simulink model "simulink_A2_Final"  (R2023a)
settings: Solver=FixedStepAuto  StartTime=0.0  StopTime=30  FixedStep=1e-3  RelTol=1e-3  EnableMultiTasking=on
undefined symbols (not defined in the file): A0, A1, D0, D1, D10, D11, D12, D13, D2, D3, D4, D5, D6, D7, D8, D9, PTA0, PTA1, PTA2, PTB2, PTB23, PTB3, PTB9, PTC16, PTC17, PTC2, PTC3, PTC4, PTD0, PTD1, PTD2, PTD3
libraries: etargetslib x24, frdmk64flib x20, dspstat3 x1
settings Model: ExtModeTrigDuration=5  Creator=Karm  LastModifiedBy=lison
settings OptimizationCC: EnhancedBackFolding=on  PassReuseOutputArgsAs=Individual arguments  ZeroExternalMemoryAtStartup=off  ZeroInternalMemoryAtStartup=off  MaxStackSize=64  OptimizeBlockOrder=speed  DifferentSizesBufferReuse=on  OptimizationCustomize=off  EfficientTunableParamExpr=on
settings DebuggingCC: ParameterPrecisionLossMsg=none  ParameterTunabilityLossMsg=error
settings HardwareCC: ProdBitPerPointer=32  ProdBitPerSizeT=32  ProdBitPerPtrDiffT=32  ProdLargestAtomicInteger=Long  ProdLargestAtomicFloat=Double  ProdWordSize=32  ProdHWDeviceType=ARM Compatible->ARM Cortex
settings SFSimCC: MATLABDynamicMemAlloc=off
settings RTWCC: Description=Embedded Coder  SystemTargetFile=ert.tlc  HardwareBoard=NXP FRDM-K64F  TLCOptions="-aInlineSetEventsForThisBaseRateFcn=TLC_FALSE -aSuppressMultiTaskScheduler=TLC_FALSE  -aRateBasedStepFcn=0"  TemplateMakefile=ert_default_tmf  Toolchain=GNU Tools for ARM Embedded Processors
settings CodeAppCC: ForceParamTrailComments=on  IgnoreCustomStorageClasses=off  OperatorAnnotations=on  SimulinkDataObjDesc=on  SFDataObjDesc=on  InsertBlockDesc=on
settings ERTTargetCC: ExtModeTransport=4  ExtModeMexFile=sendToCommService

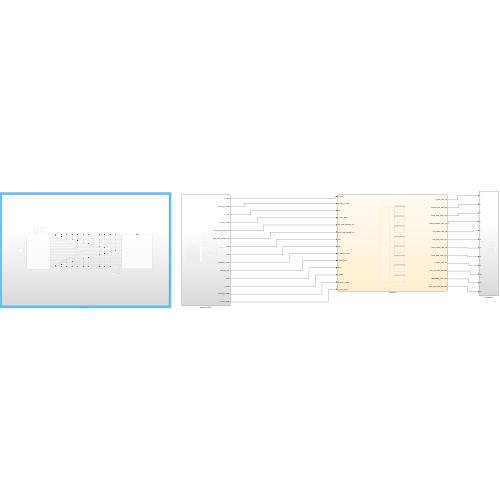
[thumbnail: Simulink's stored preview of the top-level diagram]
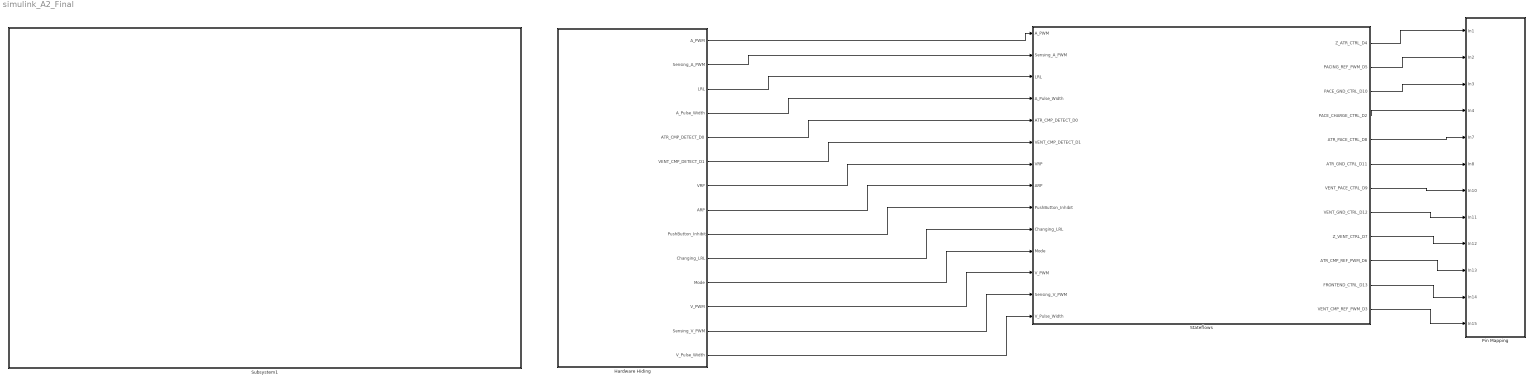
== system simulink_A2_Final ==
  Hardware Hiding : Subsystem
  Pin Mapping : Subsystem
  Stateflows : Stateflow chart  TreatAsAtomicUnit=on
      settings: PortSchema="{\"entries\":[{\"content\":{\"sides\":[{\"content\":{\"connectorIds\":[\"In1\",\"In9\",\"In2\",\"In8\",\"In3\",\"In4\",\"In5\",\"In6\",\"In7\",\"In10\",\"In11\",\"In12\",\"In13\",\"In14\"]},\"type\":\"ConnectorPlacement.EquallySpacedRectSide\",\"uuid\":\"fd7a65b5-6a9e-486c-b395-8752d247d110\"},{\"content\":{\"connectorIds\":[\"Out1\",\"Out2\",\"Out3\",\"Out4\",\"Out5\",\"Out6\",\"Out7\",\"Out8\",\"Out9\",\"Out10\",\"Out11\",\"Out12\"],\"side\":\"RIGHT\"},\"type\":\"ConnectorPlacement.EquallySpacedRectSide\",\"uuid\":\"2771a934-b7e6-4717-9d0f-b17bdbdca872\"},{\"content\":{\"side\":\"TOP\"},\"type\":\"ConnectorPlacement.EquallySpacedRectSide\",\"uuid\":\"3a68066b-1574-4876-94b5-372b67bc25b8\"}]},\"type\":\"ConnectorPlacement.EquallySpacedConnector\",\"uuid\":\"cd95133d-7553-4814-ba78-1fbdc0c00507\"}],\"packageUris\":[\"http://schema.mathworks.com/mf0/Connector/R2020b\"],\"version\":\"1.0\"}"
  Subsystem1 : Subsystem
  wires:
  Hardware Hiding/1(A_PWM) -> Stateflows/1(A_PWM)
  Hardware Hiding/2(Sensing_A_PWM) -> Stateflows/9(Sensing_A_PWM)
  Hardware Hiding/3(LRL) -> Stateflows/2(LRL)
  Hardware Hiding/4(A_Pulse_Width) -> Stateflows/8(A_Pulse_Width)
  Hardware Hiding/5(ATR_CMP_DETECT_D0) -> Stateflows/3(ATR_CMP_DETECT_D0)
  Hardware Hiding/6(VENT_CMP_DETECT_D1) -> Stateflows/4(VENT_CMP_DETECT_D1)
  Hardware Hiding/7(VRP) -> Stateflows/5(VRP)
  Hardware Hiding/8(ARP) -> Stateflows/6(ARP)
  Hardware Hiding/9(PushButton_Inhibit) -> Stateflows/7(PushButton_Inhibit)
  Stateflows/1(Z_ATR_CTRL_D4) -> Pin Mapping/1(In1)
  Stateflows/2(PACING_REF_PWM_D5) -> Pin Mapping/2(In2)
  Stateflows/3(PACE_GND_CTRL_D10) -> Pin Mapping/3(In3)
  Stateflows/4(PACE_CHARGE_CTRL_D2) -> Pin Mapping/4(In4)
  Stateflows/5(ATR_PACE_CTRL_D8) -> Pin Mapping/5(In7)
  Stateflows/6(ATR_GND_CTRL_D11) -> Pin Mapping/6(In8)
  Stateflows/7(VENT_PACE_CTRL_D9) -> Pin Mapping/7(In10)
  Stateflows/8(VENT_GND_CTRL_D12) -> Pin Mapping/8(In11)
  Stateflows/9(Z_VENT_CTRL_D7) -> Pin Mapping/9(In12)
  Stateflows/10(ATR_CMP_REF_PWM_D6) -> Pin Mapping/10(In13)
  Stateflows/11(FRONTEND_CTRL_D13) -> Pin Mapping/11(In14)
  Stateflows/12(VENT_CMP_REF_PWM_D3) -> Pin Mapping/12(In15)
  Hardware Hiding/10(Changing_LRL) -> Stateflows/10(Changing_LRL)
  Hardware Hiding/11(Mode) -> Stateflows/11(Mode)
  Hardware Hiding/12(V_PWM) -> Stateflows/12(V_PWM)
  Hardware Hiding/13(Sensing_V_PWM) -> Stateflows/13(Sensing_V_PWM)
  Hardware Hiding/14(V_Pulse_Width) -> Stateflows/14(V_Pulse_Width)

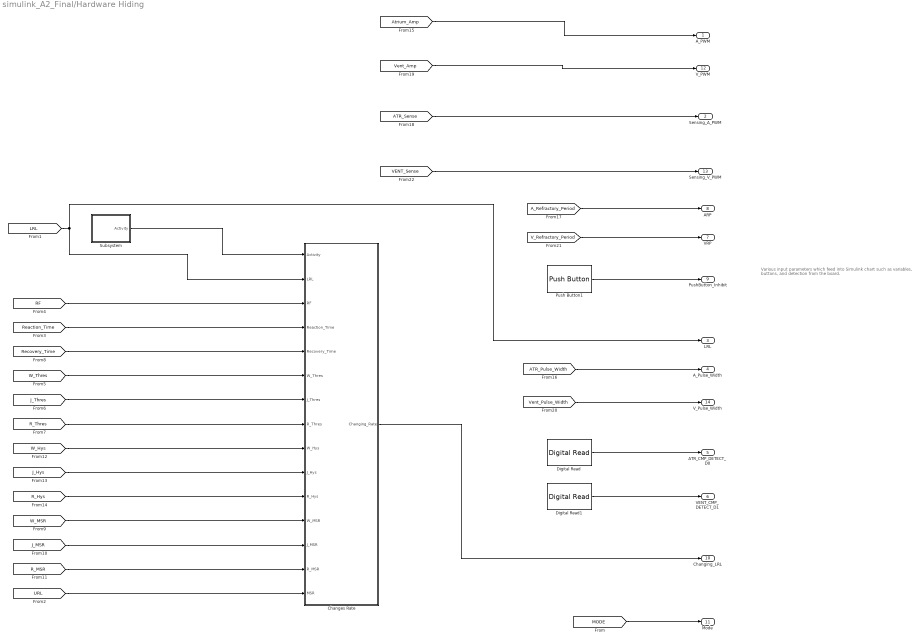
== system simulink_A2_Final/Hardware Hiding ==
  note: Various input parameters which feed into
      | Simulink chart such as variables, buttons, and
      | detection from the board.
  Changes Rate : Stateflow chart  TreatAsAtomicUnit=on
  Digital Read : frdmk64flib/Digital Read  Whichpin=PTC16 (D0)  SampleTime=-1
  Digital Read1 : frdmk64flib/Digital Read  Whichpin=PTC17 (D1)  SampleTime=-1
  Push Button1 : frdmk64flib/Push Button  Whichswitch=SW3  SampleTime1=-1
  Subsystem : Subsystem
  A_PWM : Outport  OutDataTypeStr=single
  Sensing_A_PWM : Outport  Port=2  OutDataTypeStr=single
  LRL : Outport  Port=3  OutDataTypeStr=uint16
  A_Pulse_Width : Outport  Port=4  OutDataTypeStr=uint16
  ATR_CMP_DETECT_D0 : Outport  Port=5
  VENT_CMP_DETECT_D1 : Outport  Port=6
  VRP : Outport  Port=7  OutDataTypeStr=uint16
  ARP : Outport  Port=8  OutDataTypeStr=uint16
  PushButton_Inhibit : Outport  Port=9
  Changing_LRL : Outport  Port=10  OutDataTypeStr=uint16
  Mode : Outport  Port=11  OutDataTypeStr=uint8
  V_PWM : Outport  Port=12  OutDataTypeStr=single
  Sensing_V_PWM : Outport  Port=13
  V_Pulse_Width : Outport  Port=14  OutDataTypeStr=uint16
  wires:
  Push Button1/1 -> PushButton_Inhibit/1
  [V_Refractory_Period] -> VRP/1
  [A_Refractory_Period] -> ARP/1
  [LRL] -> LRL/1, Changes Rate/2(LRL)
  [ATR_Pulse_Width] -> A_Pulse_Width/1
  Digital Read/1 -> ATR_CMP_DETECT_D0/1
  Digital Read1/1 -> VENT_CMP_DETECT_D1/1
  [W_Thres] -> Changes Rate/6(W_Thres)
  [RF] -> Changes Rate/3(RF)
  [Recovery_Time] -> Changes Rate/5(Recovery_Time)
  [J_Thres] -> Changes Rate/7(J_Thres)
  [R_Thres] -> Changes Rate/8(R_Thres)
  [W_Hys] -> Changes Rate/9(W_Hys)
  [J_Hys] -> Changes Rate/10(J_Hys)
  [R_Hys] -> Changes Rate/11(R_Hys)
  [W_MSR] -> Changes Rate/12(W_MSR)
  [J_MSR] -> Changes Rate/13(J_MSR)
  [R_MSR] -> Changes Rate/14(R_MSR)
  Subsystem/1(Activity) -> Changes Rate/1(Activity)
  [Reaction_Time] -> Changes Rate/4(Reaction_Time)
  Changes Rate/1(Changing_Rate) -> Changing_LRL/1
  [URL] -> Changes Rate/15(MSR)
  [MODE] -> Mode/1
  [Vent_Pulse_Width] -> V_Pulse_Width/1
  [VENT_Sense] -> Sensing_V_PWM/1
  [ATR_Sense] -> Sensing_A_PWM/1
  [Vent_Amp] -> V_PWM/1
  [Atrium_Amp] -> A_PWM/1

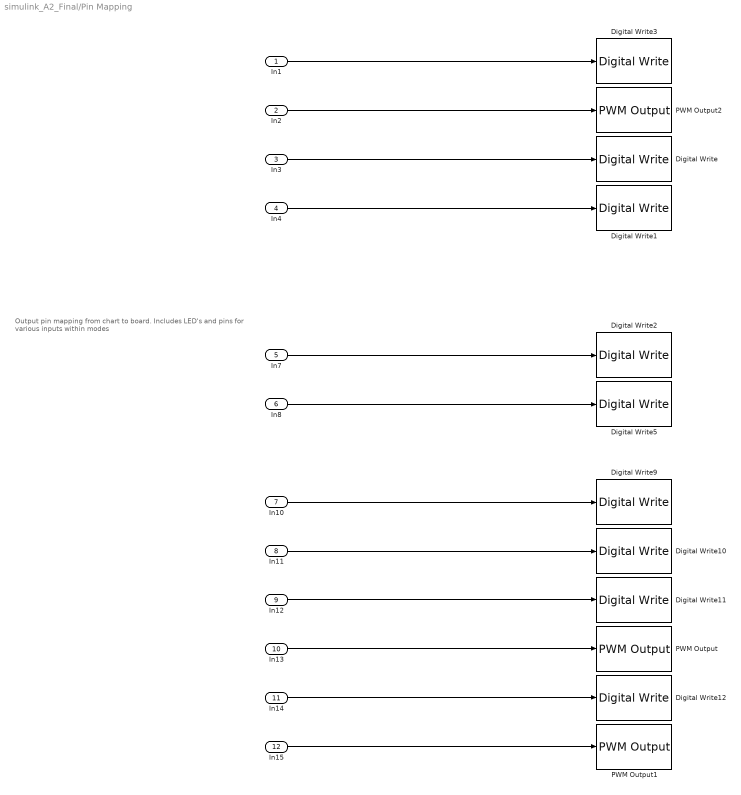
== system simulink_A2_Final/Pin Mapping ==
  note: Output pin mapping from chart to board.
      | Includes LED's and pins for various
      | inputs within modes
  In1 : Inport
  In2 : Inport  Port=2
  In3 : Inport  Port=3
  In4 : Inport  Port=4
  In7 : Inport  Port=5
  In8 : Inport  Port=6
  In10 : Inport  Port=7
  In11 : Inport  Port=8
  In12 : Inport  Port=9
  In13 : Inport  Port=10
  In14 : Inport  Port=11
  In15 : Inport  Port=12
  Digital Write : frdmk64flib/Digital Write  Whichpin=PTD0 (D10)
  Digital Write1 : frdmk64flib/Digital Write  Whichpin=PTB9 (D2)
  Digital Write10 : frdmk64flib/Digital Write  Whichpin=PTD3 (D12)
  Digital Write11 : frdmk64flib/Digital Write  Whichpin=PTC3 (D7)
  Digital Write12 : frdmk64flib/Digital Write  Whichpin=PTD1 (D13)
  Digital Write2 : frdmk64flib/Digital Write  Whichpin=PTA0 (D8)
  Digital Write3 : frdmk64flib/Digital Write  Whichpin=PTB23 (D4)
  Digital Write5 : frdmk64flib/Digital Write  Whichpin=PTD2 (D11)
  Digital Write9 : frdmk64flib/Digital Write  Whichpin=PTC4 (D9)
  PWM Output : frdmk64flib/PWM Output  Whichpin=PTC2 (D6)  InitialFrequency=2000  InitialDutyCycle=0
  PWM Output1 : frdmk64flib/PWM Output  Whichpin=PTA1 (D3)  InitialFrequency=2000  InitialDutyCycle=0
  PWM Output2 : frdmk64flib/PWM Output  Whichpin=PTA2 (D5)  InitialFrequency=2000  InitialDutyCycle=0
  wires:
  In1/1 -> Digital Write3/1
  In2/1 -> PWM Output2/1
  In4/1 -> Digital Write1/1
  In8/1 -> Digital Write5/1
  In7/1 -> Digital Write2/1
  In3/1 -> Digital Write/1
  In12/1 -> Digital Write11/1
  In10/1 -> Digital Write9/1
  In11/1 -> Digital Write10/1
  In13/1 -> PWM Output/1
  In15/1 -> PWM Output1/1
  In14/1 -> Digital Write12/1

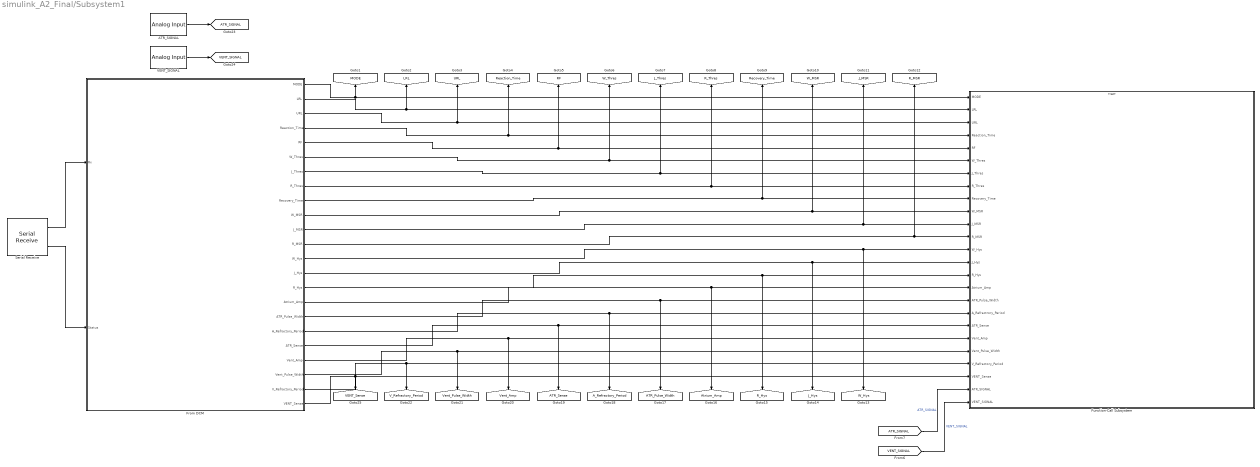
== system simulink_A2_Final/Subsystem1 ==
  ATR_SIGNAL : frdmk64flib/Analog Input  Whichpin=PTB2 (A0)  SampleTime=-1
  From DCM : Stateflow chart  TreatAsAtomicUnit=on
      settings: PortSchema="{\"entries\":[{\"content\":{\"sides\":[{\"content\":{\"connectorIds\":[\"In1\",\"In2\"]},\"type\":\"ConnectorPlacement.EquallySpacedRectSide\",\"uuid\":\"cf186c72-5509-48fa-91bf-627d929b9ac9\"},{\"content\":{\"connectorIds\":[\"Out3\",\"Out1\",\"Out2\",\"Out4\",\"Out5\",\"Out6\",\"Out7\",\"Out8\",\"Out9\",\"Out10\",\"Out11\",\"Out12\",\"Out13\",\"Out14\",\"Out15\",\"Out16\",\"Out17\",\"Out18\",\"Out19\",\"Out20\",\"Out21\",\"Out22\",\"Out23\"],\"side\":\"RIGHT\"},\"type\":\"ConnectorPlacement.EquallySpacedRectSide\",\"uuid\":\"f11b7b65-e2af-422d-8d59-d5e19782ba77\"},{\"content\":{\"side\":\"TOP\"},\"type\":\"ConnectorPlacement.EquallySpacedRectSide\",\"uuid\":\"83f5ca47-954b-473f-a694-ccb4a0a9db86\"},{\"content\":{\"side\":\"BOTTOM\"},\"type\":\"ConnectorPlacement.EquallySpacedRectSide\",\"uuid\":\"1b259bf9-85ed-487d-ae78-9bbf0cb8bebe\"}]},\"type\":\"ConnectorPlacement.EquallySpacedConnector\",\"uuid\":\"33095ea8-75ce-40a2-933c-32919530d49f\"}],\"packageUris\":[\"http://schema.mathworks.com/mf0/Connector/R2020b\"],\"version\":\"1.0\"}"
  Function-Call Subsystem : Subsystem  TreatAsAtomicUnit=on
  Serial Receive : frdmk64flib/Serial Receive  SCIModule=0  Baudrate=uint32(9600)  Parity=None  StopBits=1  HardwareFlowControl=None  ByteOrder=LittleEndian  DataType=uint8  DataLength=91  BlockingMode=off  OutputStatus=on  SampleTime=-1
  VENT_SIGNAL : frdmk64flib/Analog Input  Whichpin=PTB3 (A1)  SampleTime=-1
  tag scope: ATR_Pulse_Width=global, ATR_SIGNAL=global, ATR_Sense=global, A_Refractory_Period=global, Atrium_Amp=global, J_Hys=global, J_MSR=global, J_Thres=global, LRL=global, MODE=global, RF=global, R_Hys=global, R_MSR=global, R_Thres=global, Reaction_Time=global, Recovery_Time=global, URL=global, VENT_SIGNAL=global, VENT_Sense=global, V_Refractory_Period=global, Vent_Amp=global, Vent_Pulse_Width=global, W_Hys=global, W_MSR=global, W_Thres=global
  wires:
  Serial Receive/2 -> From DCM/2(Status)
  Serial Receive/1 -> From DCM/1(Rx)
  From DCM/3(MODE) -> Function-Call Subsystem/1(MODE), [MODE]
  From DCM/1(LRL) -> Function-Call Subsystem/2(LRL), [LRL]
  From DCM/2(URL) -> Function-Call Subsystem/3(URL), [URL]
  From DCM/4(Reaction_Time) -> Function-Call Subsystem/4(Reaction_Time), [Reaction_Time]
  From DCM/5(RF) -> Function-Call Subsystem/5(RF), [RF]
  From DCM/6(W_Thres) -> Function-Call Subsystem/6(W_Thres), [W_Thres]
  From DCM/7(J_Thres) -> Function-Call Subsystem/7(J_Thres), [J_Thres]
  From DCM/8(R_Thres) -> Function-Call Subsystem/8(R_Thres), [R_Thres]
  From DCM/9(Recovery_Time) -> Function-Call Subsystem/9(Recovery_Time), [Recovery_Time]
  From DCM/10(W_MSR) -> Function-Call Subsystem/10(W_MSR), [W_MSR]
  From DCM/11(J_MSR) -> Function-Call Subsystem/11(J_MSR), [J_MSR]
  From DCM/12(R_MSR) -> Function-Call Subsystem/12(R_MSR), [R_MSR]
  From DCM/13(W_Hys) -> Function-Call Subsystem/13(W_Hys), [W_Hys]
  From DCM/14(J_Hys) -> Function-Call Subsystem/14(J_Hys), [J_Hys]
  From DCM/15(R_Hys) -> Function-Call Subsystem/15(R_Hys), [R_Hys]
  From DCM/16(Atrium_Amp) -> Function-Call Subsystem/16(Atrium_Amp), [Atrium_Amp]
  From DCM/17(ATR_Pulse_Width) -> Function-Call Subsystem/17(ATR_Pulse_Width), [ATR_Pulse_Width]
  From DCM/18(A_Refractory_Period) -> Function-Call Subsystem/18(A_Refractrory_Period), [A_Refractory_Period]
  From DCM/19(ATR_Sense) -> Function-Call Subsystem/19(ATR_Sense), [ATR_Sense]
  From DCM/21(Vent_Pulse_Width) -> Function-Call Subsystem/21(Vent_Pulse_Width), [Vent_Pulse_Width]
  From DCM/22(V_Refractory_Period) -> Function-Call Subsystem/22(V_Refractory_Period), [V_Refractory_Period]
  From DCM/23(VENT_Sense) -> Function-Call Subsystem/23(VENT_Sense), [VENT_Sense]
  ATR_SIGNAL/1 -> [ATR_SIGNAL]
  VENT_SIGNAL/1 -> [VENT_SIGNAL]
  From DCM/20(Vent_Amp) -> Function-Call Subsystem/20(Vent_Amp), [Vent_Amp]
  [ATR_SIGNAL] -> Function-Call Subsystem/24(ATR_SIGNAL)  "ATR_SIGNAL"
  [VENT_SIGNAL] -> Function-Call Subsystem/25(VENT_SIGNAL)  "VENT_SIGNAL"

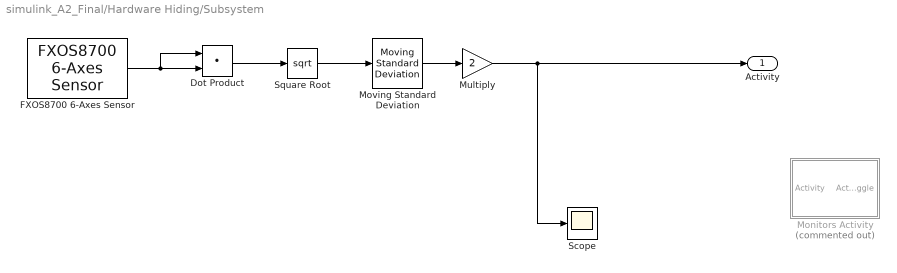
== system simulink_A2_Final/Hardware Hiding/Subsystem ==
  Dot Product : DotProduct  OutDataTypeStr=Inherit: Inherit via internal rule
  FXOS8700 6-Axes Sensor : frdmk64flib/FXOS8700 6-Axes Sensor  Activesensor=Accelerometer only  ODR=800Hz  HybridODR=400Hz  Accelfullrange=-4g to +4g  SampleTime=-1
  Monitors Activity : Stateflow chart  Commented=on  TreatAsAtomicUnit=on
  Moving Standard Deviation : dspstat3/Moving Standard Deviation  Method=Sliding window  ForgettingFactorPort=off  SpecifyWindowLength=on  WindowLength=4  OverlapLength=3  AllowArbitraryInputLength=off  ForgettingFactor=0.9  SimulateUsing=Code generation
  Multiply : Gain  Gain=2
  Scope : Scope
  Square Root : Sqrt
  Activity : Outport
  wires:
  Square Root/1 -> Moving Standard Deviation/1
  Moving Standard Deviation/1 -> Multiply/1
  Dot Product/1 -> Square Root/1
  FXOS8700 6-Axes Sensor/1 -> Dot Product/2, Dot Product/1
  Multiply/1 -> Scope/1, Activity/1

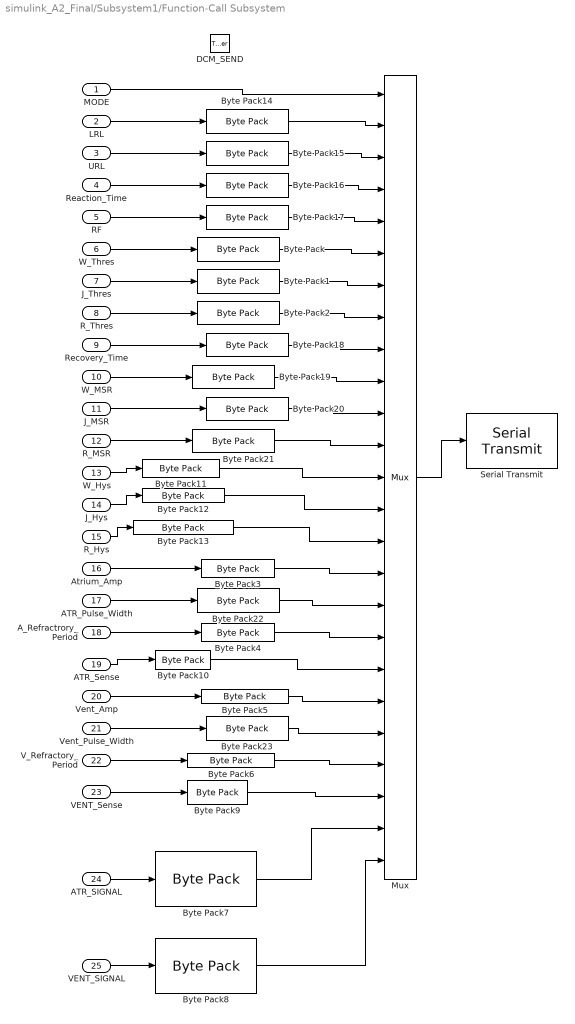
== system simulink_A2_Final/Subsystem1/Function-Call Subsystem ==
  MODE : Inport  OutDataTypeStr=uint8
  LRL : Inport  Port=2  OutDataTypeStr=uint16
  URL : Inport  Port=3  OutDataTypeStr=uint16
  Reaction_Time : Inport  Port=4  OutDataTypeStr=uint16
  RF : Inport  Port=5  OutDataTypeStr=uint16
  W_Thres : Inport  Port=6  OutDataTypeStr=double
  J_Thres : Inport  Port=7  OutDataTypeStr=double
  R_Thres : Inport  Port=8  OutDataTypeStr=double
  Recovery_Time : Inport  Port=9  OutDataTypeStr=uint16
  W_MSR : Inport  Port=10  OutDataTypeStr=uint16
  J_MSR : Inport  Port=11  OutDataTypeStr=uint16
  R_MSR : Inport  Port=12  OutDataTypeStr=uint16
  W_Hys : Inport  Port=13  OutDataTypeStr=double
  J_Hys : Inport  Port=14  OutDataTypeStr=double
  R_Hys : Inport  Port=15  OutDataTypeStr=double
  Atrium_Amp : Inport  Port=16  OutDataTypeStr=single
  ATR_Pulse_Width : Inport  Port=17  OutDataTypeStr=uint16
  A_Refractrory_Period : Inport  Port=18  OutDataTypeStr=uint16
  ATR_Sense : Inport  Port=19  OutDataTypeStr=single
  Vent_Amp : Inport  Port=20  OutDataTypeStr=single
  Vent_Pulse_Width : Inport  Port=21  OutDataTypeStr=uint16
  V_Refractory_Period : Inport  Port=22  OutDataTypeStr=uint16
  VENT_Sense : Inport  Port=23  OutDataTypeStr=single
  ATR_SIGNAL : Inport  Port=24  OutDataTypeStr=double
  VENT_SIGNAL : Inport  Port=25  OutDataTypeStr=double
  DCM_SEND : TriggerPort  TriggerType=function-call  IsSimulinkFunction=on  FunctionName=DCM_SEND  VariantControl=(inherit)
  Byte Pack{,1..2,7..8,11..13} (8 alike) : etargetslib/Byte Pack  datatypes={'double'}  byteAlign=1
  Byte Pack{3,5,9..10} (4 alike) : etargetslib/Byte Pack  datatypes={'single'}  byteAlign=1
  Byte Pack{4,6,14..23} (12 alike) : etargetslib/Byte Pack  datatypes={'uint16'}  byteAlign=1
  Mux : Mux  Inputs=25
  Serial Transmit : frdmk64flib/Serial Transmit  SCIModule=0  Baudrate=uint32(9600)  Parity=None  StopBits=1  HardwareFlowControl=None  ByteOrder=LittleEndian  BlockingMode=on  OutputStatus=off
  wires:
  MODE/1 -> Mux/1
  Reaction_Time/1 -> Byte Pack16/1
  RF/1 -> Byte Pack17/1
  W_Thres/1 -> Byte Pack/1
  Byte Pack/1 -> Mux/6
  J_Thres/1 -> Byte Pack1/1
  Byte Pack1/1 -> Mux/7
  Recovery_Time/1 -> Byte Pack18/1
  R_Thres/1 -> Byte Pack2/1
  Byte Pack2/1 -> Mux/8
  W_MSR/1 -> Byte Pack19/1
  J_MSR/1 -> Byte Pack20/1
  R_MSR/1 -> Byte Pack21/1
  Atrium_Amp/1 -> Byte Pack3/1
  ATR_Pulse_Width/1 -> Byte Pack22/1
  Byte Pack3/1 -> Mux/16
  A_Refractrory_Period/1 -> Byte Pack4/1
  Byte Pack4/1 -> Mux/18
  Vent_Amp/1 -> Byte Pack5/1
  Byte Pack5/1 -> Mux/20
  Vent_Pulse_Width/1 -> Byte Pack23/1
  V_Refractory_Period/1 -> Byte Pack6/1
  Byte Pack6/1 -> Mux/22
  Mux/1 -> Serial Transmit/1
  ATR_SIGNAL/1 -> Byte Pack7/1
  Byte Pack7/1 -> Mux/24
  VENT_SIGNAL/1 -> Byte Pack8/1
  Byte Pack8/1 -> Mux/25
  VENT_Sense/1 -> Byte Pack9/1
  Byte Pack9/1 -> Mux/23
  ATR_Sense/1 -> Byte Pack10/1
  Byte Pack10/1 -> Mux/19
  W_Hys/1 -> Byte Pack11/1
  Byte Pack11/1 -> Mux/13
  J_Hys/1 -> Byte Pack12/1
  Byte Pack12/1 -> Mux/14
  R_Hys/1 -> Byte Pack13/1
  Byte Pack13/1 -> Mux/15
  LRL/1 -> Byte Pack14/1
  Byte Pack14/1 -> Mux/2
  URL/1 -> Byte Pack15/1
  Byte Pack15/1 -> Mux/3
  Byte Pack16/1 -> Mux/4
  Byte Pack17/1 -> Mux/5
  Byte Pack18/1 -> Mux/9
  Byte Pack19/1 -> Mux/10
  Byte Pack20/1 -> Mux/11
  Byte Pack21/1 -> Mux/12
  Byte Pack22/1 -> Mux/17
  Byte Pack23/1 -> Mux/21

== stateflow chart simulink_A2_Final/Hardware Hiding/Subsystem/Monitors Activity ==
  state entry
    if Activity > 1.0
    Act_Toggle = true;
    else
    Act_Toggle = false;
    end
  (default) -> entry
  data: Activity input; Act_Toggle output

== stateflow chart simulink_A2_Final/Stateflows ==
  state Start
  state VOO
    state Charging
      % parameters laid out by documentation for Charging
      entry:
      PACING_REF_PWM_D5 = (V_PWM/5)*100;
      PACE_GND_CTRL_D10 = 1;
      VENT_GND_CTRL_D12 = 1;
      PACE_CHARGE_CTRL_D2 = 1;
      Z_VENT_CTRL_D7 = 0;
      VENT_PACE_CTRL_D9 = 0;
      Pulse_Period = (60000/LRL);
    state Pacing
      % parameters laid out by documentation for Pacing
      entry:
      PACING_REF_PWM_D5 = (V_PWM/5)*100;
      VENT_PACE_CTRL_D9 = 1;
      VENT_GND_CTRL_D12 = 0;
      PACE_CHARGE_CTRL_D2 = 0;
      PACE_GND_CTRL_D10 = 1;
      Z_VENT_CTRL_D7 = 0;
    note: Ventricular pacing, no sensing
    (default) -> VOO.Charging
    VOO.Charging -> VOO.Pacing : [after(Pulse_Period-V_Pulse_Width,msec)]
    VOO.Pacing -> VOO.Charging : [after(V_Pulse_Width,msec)]
  state VVI
    note: Ventricular pacing, ventricular sensing, sensed intrinsic signal inhibits ventricular pacing
    state Pacing2
      % parameters laid out by documentation for Pacing
      entry:
      PACE_CHARGE_CTRL_D2 = 0;
      PACE_GND_CTRL_D10 = 1;
      Z_VENT_CTRL_D7 = 0;
      VENT_GND_CTRL_D12 = 0;
      VENT_PACE_CTRL_D9 = 1;
    state Charging2
      % parameters laid out by documentation for Charging
      entry:
      FRONTEND_CTRL_D13 = 1;
      VENT_CMP_REF_PWM_D3 = (Sensing_V_PWM/5)*100;
      PACING_REF_PWM_D5 = (V_PWM/5)*100;
      VENT_PACE_CTRL_D9 = 0;
      PACE_CHARGE_CTRL_D2 = 1;
      PACE_GND_CTRL_D10 = 1;
      Z_VENT_CTRL_D7 = 0;
      VENT_GND_CTRL_D12 = 1;
      Pulse_Period = (60000/LRL);
    state Refractor_and_Sensing
    (default) -> VVI.Charging2
    VVI.Pacing2 -> VVI.Charging2 : [after(V_Pulse_Width,msec)]
    VVI.Refractor_and_Sensing -> VVI.Pacing2 [order 2] : after(Pulse_Period-VRP-V_Pulse_Width,msec)[VENT_CMP_DETECT_D1 == 0 & PushButton_Inhibit == false]
    VVI.Charging2 -> VVI.Refractor_and_Sensing : after(VRP,msec)
    VVI.Refractor_and_Sensing -> VVI.Charging2 [order 1] : [VENT_CMP_DETECT_D1 == 1 | PushButton_Inhibit == true]
  state AOO
    note: Atrial pacing, no sensing
    state Charging1
      % parameters laid out by documentation for Charging
      entry:
      PACING_REF_PWM_D5 = (A_PWM/5)*100;
      PACE_CHARGE_CTRL_D2 = 1;
      ATR_PACE_CTRL_D8 = 0;
      PACE_GND_CTRL_D10 = 1;
      ATR_GND_CTRL_D11 = 1;
      Z_ATR_CTRL_D4 = 0;
      Pulse_Period = (60000/LRL);
    state Pacing1
      % parameters laid out by documentation for Pacing
      entry:
      PACING_REF_PWM_D5 = (A_PWM/5)*100;
      PACE_CHARGE_CTRL_D2 = 0;
      PACE_GND_CTRL_D10 = 1;
      ATR_PACE_CTRL_D8 = 1;
      ATR_GND_CTRL_D11 = 0;
      Z_ATR_CTRL_D4 = 0;
    (default) -> AOO.Charging1
    AOO.Charging1 -> AOO.Pacing1 : [after(Pulse_Period-A_Pulse_Width,msec)]
    AOO.Pacing1 -> AOO.Charging1 : [after(A_Pulse_Width,msec)]
  state AAI
    state Pacing3
      % parameters laid out by documentation for Pacing
      entry:
      PACING_REF_PWM_D5 = (A_PWM/5)*100;
      PACE_CHARGE_CTRL_D2=0;
      ATR_PACE_CTRL_D8= 1;
      ATR_GND_CTRL_D11= 0;
      PACE_GND_CTRL_D10=1;
      Z_ATR_CTRL_D4=0;
    state Charging3
      % parameters laid out by documentation for Charging
      entry:
      PACING_REF_PWM_D5 = (A_PWM/5)*100;
      PACE_CHARGE_CTRL_D2=1;
      ATR_PACE_CTRL_D8= 0;
      ATR_GND_CTRL_D11= 1;
      PACE_GND_CTRL_D10=1;
      Z_ATR_CTRL_D4=0;
      FRONTEND_CTRL_D13 = 1;
      ATR_CMP_REF_PWM_D6 = (Sensing_A_PWM/5)*100;
      Pulse_Period = (60000/LRL);
    state Refractor_and_Sensing
    note: Atrial pacing, atrial sensing, sensed intrinsic signal inhibits atrial pacing
    (default) -> AAI.Charging3
    AAI.Refractor_and_Sensing -> AAI.Charging3 [order 1] : [ATR_CMP_DETECT_D0 == 1 | PushButton_Inhibit == true]
    AAI.Refractor_and_Sensing -> AAI.Pacing3 [order 2] : after(Pulse_Period-ARP-A_Pulse_Width,msec)[ATR_CMP_DETECT_D0 == 0 & PushButton_Inhibit == false]
    AAI.Charging3 -> AAI.Refractor_and_Sensing : after(ARP, msec)
    AAI.Pacing3 -> AAI.Charging3 : after(A_Pulse_Width,msec)
  state VOOR
    state Charging
      % parameters laid out by documentation for Charging
      entry:
      PACING_REF_PWM_D5 = (V_PWM/5)*100;
      PACE_CHARGE_CTRL_D2 = 1;
      VENT_PACE_CTRL_D9 = 0;
      PACE_GND_CTRL_D10 = 1;
      Z_VENT_CTRL_D7 = 0;
      VENT_GND_CTRL_D12 = 1;
      Changing_Rate = (60000/Changing_LRL);
    state Pacing
      % parameters laid out by documentation for Pacing
      entry:
      PACING_REF_PWM_D5 = (V_PWM/5)*100;
      PACE_CHARGE_CTRL_D2 = 0;
      PACE_GND_CTRL_D10 = 1;
      Z_VENT_CTRL_D7 = 0;
      VENT_GND_CTRL_D12 = 0;
      VENT_PACE_CTRL_D9 = 1;
    note: Ventricular pacing, no sensing; Rate Adaptive Mode
    (default) -> VOOR.Charging
    VOOR.Charging -> VOOR.Pacing : [after(Changing_Rate-V_Pulse_Width,msec)]
    VOOR.Pacing -> VOOR.Charging : [after(V_Pulse_Width,msec)]
  state VVIR
    note: Ventricular pacing, ventricular sensing, sensed intrinsic signal inhibits ventricular pacing, Rate Adaptive Mode
    state Pacing2
      % parameters laid out by documentation for Pacing
      entry:
      PACE_CHARGE_CTRL_D2 = 0;
      PACE_GND_CTRL_D10 = 1;
      Z_VENT_CTRL_D7 = 0;
      VENT_GND_CTRL_D12 = 0;
      VENT_PACE_CTRL_D9 = 1;
    state Charging2
      % parameters laid out by documentation for Charging
      entry:
      FRONTEND_CTRL_D13 = 1;
      VENT_CMP_REF_PWM_D3 = (Sensing_V_PWM/5)*100;
      PACING_REF_PWM_D5 = (V_PWM/5)*100;
      VENT_PACE_CTRL_D9 = 0;
      PACE_CHARGE_CTRL_D2 = 1;
      PACE_GND_CTRL_D10 = 1;
      Z_VENT_CTRL_D7 = 0;
      VENT_GND_CTRL_D12 = 1;
      Changing_Rate = (60000/Changing_LRL);
    state Refractor_and_Sensing
    (default) -> VVIR.Charging2
    VVIR.Pacing2 -> VVIR.Charging2 : [after(V_Pulse_Width,msec)]
    VVIR.Refractor_and_Sensing -> VVIR.Pacing2 [order 2] : after(Changing_Rate-VRP-V_Pulse_Width,msec)[VENT_CMP_DETECT_D1 == 0 & PushButton_Inhibit == false]
    VVIR.Charging2 -> VVIR.Refractor_and_Sensing : after(VRP,msec)
    VVIR.Refractor_and_Sensing -> VVIR.Charging2 [order 1] : [VENT_CMP_DETECT_D1 == 1 | PushButton_Inhibit == true]
  state AOOR
    note: Atrial pacing, no sensing; Rate Adaptive Mode
    state Charging1
      % parameters laid out by documentation for Charging
      entry:
      PACING_REF_PWM_D5 = (A_PWM/5)*100;
      PACE_CHARGE_CTRL_D2 = 1;
      ATR_PACE_CTRL_D8 = 0;
      PACE_GND_CTRL_D10 = 1;
      ATR_GND_CTRL_D11 = 1;
      Z_ATR_CTRL_D4 = 0;
      Changing_Rate = (60000/Changing_LRL);
    state Pacing1
      % parameters laid out by documentation for Pacing
      entry:
      PACING_REF_PWM_D5 = (A_PWM/5)*100;
      PACE_CHARGE_CTRL_D2 = 0;
      PACE_GND_CTRL_D10 = 1;
      ATR_PACE_CTRL_D8 = 1;
      ATR_GND_CTRL_D11 = 0;
      Z_ATR_CTRL_D4 = 0;
    (default) -> AOOR.Charging1
    AOOR.Charging1 -> AOOR.Pacing1 : [after(Changing_Rate-A_Pulse_Width,msec)]
    AOOR.Pacing1 -> AOOR.Charging1 : [after(A_Pulse_Width,msec)]
  state AAIR
    state Charging3
      % parameters laid out by documentation for Charging
      entry:
      PACING_REF_PWM_D5 = (A_PWM/5)*100;
      PACE_CHARGE_CTRL_D2=1;
      ATR_PACE_CTRL_D8= 0;
      ATR_GND_CTRL_D11= 1;
      PACE_GND_CTRL_D10=1;
      Z_ATR_CTRL_D4=0;
      FRONTEND_CTRL_D13 = 1;
      ATR_CMP_REF_PWM_D6 = (Sensing_A_PWM/5)*100;
      Changing_Rate = (60000/Changing_LRL);
    state Pacing3
      % parameters laid out by documentation for Pacing
      entry:
      PACING_REF_PWM_D5 = (A_PWM/5)*100;
      PACE_CHARGE_CTRL_D2=0;
      ATR_PACE_CTRL_D8= 1;
      ATR_GND_CTRL_D11= 0;
      PACE_GND_CTRL_D10=1;
      Z_ATR_CTRL_D4=0;
    state Refractor_and_Sensing
    note: Atrial pacing, atrial sensing, sensed intrinsic signal inhibits atrial pacing, Rate Adaptive Mode
    (default) -> AAIR.Charging3
    AAIR.Refractor_and_Sensing -> AAIR.Charging3 [order 1] : [ATR_CMP_DETECT_D0 == 1 | PushButton_Inhibit == true]
    AAIR.Refractor_and_Sensing -> AAIR.Pacing3 [order 2] : after(Changing_Rate-ARP-A_Pulse_Width,msec)[ATR_CMP_DETECT_D0 == 0 & PushButton_Inhibit == false]
    AAIR.Charging3 -> AAIR.Refractor_and_Sensing : after(ARP, msec)
    AAIR.Pacing3 -> AAIR.Charging3 : after(A_Pulse_Width,msec)
  (default) -> Start
  Start -> VOO [order 1] : [Mode == 1]
  VOO -> Start : [Mode ~= 1]
  Start -> VVI [order 2] : [Mode == 2]
  VVI -> Start : [Mode ~= 2]
  Start -> AOO [order 3] : [Mode == 3]
  AOO -> Start : [Mode ~= 3]
  Start -> AAI [order 4] : [Mode == 4]
  AAI -> Start : [Mode ~= 4]
  Start -> VOOR [order 5] : [Mode == 5]
  VOOR -> Start : [Mode ~= 5]
  Start -> VVIR [order 6] : [Mode == 6]
  VVIR -> Start : [Mode ~= 6]
  Start -> AOOR [order 7] : [Mode == 7]
  AOOR -> Start : [Mode ~= 7]
  Start -> AAIR [order 8] : [Mode == 8]
  AAIR -> Start : [Mode ~= 8]
  data: A_PWM input single; LRL input uint16; ATR_CMP_DETECT_D0 input; VENT_CMP_DETECT_D1 input; VRP input uint16; ARP input uint16; PushButton_Inhibit input; A_Pulse_Width input uint16; Sensing_A_PWM input single; Z_ATR_CTRL_D4 output; PACING_REF_PWM_D5 output; PACE_GND_CTRL_D10 output; PACE_CHARGE_CTRL_D2 output; ATR_PACE_CTRL_D8 output; ATR_GND_CTRL_D11 output; VENT_PACE_CTRL_D9 output; VENT_GND_CTRL_D12 output; Z_VENT_CTRL_D7 output; ATR_CMP_REF_PWM_D6 output; FRONTEND_CTRL_D13 output; VENT_CMP_REF_PWM_D3 output; Changing_LRL input uint16; Response_Period local; Mode input uint8; V_PWM input single; Sensing_V_PWM input; V_Pulse_Width input uint16; Pulse_Period local uint16; Changing_Rate local uint16

== stateflow chart simulink_A2_Final/Hardware Hiding/Changes Rate ==
  state Changes_Accelerations1
    entry:
    if Activity < W_Thres %walking
    Thres = W_Thres;
    Hys = W_Hys;
    Accel = W_Accel;
    elseif Activity >= J_Thres && Activity < R_Thres %jogging
    Thres = J_Thres;
    Hys = J_Hys;
    Accel = J_Accel;
    elseif Activity >= R_Thres %running
    Thres = R_Thres;
    Hys = R_Hys;
    Accel = R_Accel;
    end
  state Changes_Accelerations
    entry:
    if Activity < W_Thres %walking
    Thres = W_Thres;
    Hys = W_Hys;
    Accel = W_Accel;
    elseif Activity >= J_Thres && Activity < R_Thres %jogging
    Thres = J_Thres;
    Hys = J_Hys;
    Accel = J_Accel;
    elseif Activity >= R_Thres %running
    Thres = R_Thres;
    Hys = R_Hys;
    Accel = R_Accel;
    end
  state Starting_State
    entry:
    Changing_Rate = LRL;
  state Walking_Accel
    entry:
    Changing_Rate = Changing_Rate + Accel;
  state Steady
    entry:
    Changing_Rate = MSR;
  state Changes_To_Deceleration
    entry:
    if Hys == W_Hys
    Decel = W_Decel;
    elseif Hys == J_Hys
    Decel = J_Decel;
    elseif Hys == R_Hys
    Decel == R_Decel;
    end
  state Changes_To_Acceleration
    entry:
    if Thres == W_Thres
    Accel = W_Accel;
    elseif Thres == J_Thres
    Accel = J_Accel;
    elseif Thres == R_Thres
    Accel == R_Accel;
    end
  state Walking_Decel
    entry:
    Changing_Rate = Changing_Rate - Decel;
  state Changes_Decelerations
    entry:
    if Activity < W_Hys %walking
    Thres = W_Thres;
    Hys = W_Hys;
    Decel = W_Decel;
    elseif Activity >= W_Thres && Activity < J_Hys %jogging
    Thres = J_Thres;
    Hys = J_Hys;
    Decel = J_Decel;
    elseif Activity > J_Thres && Activity < R_Hys %running
    Thres = R_Thres;
    Hys = R_Hys;
    Decel = R_Decel;
    end
  (default) -> Starting_State : {
      | W_Accel = ceil((W_MSR - LRL)*RF/(Reaction_Time*10/60))
      | W_Decel = ceil((W_MSR - LRL)*(RF/8)/Recovery_Time)
      | J_Accel = ceil((J_MSR - LRL)*RF/(Reaction_Time*10/60))
      | J_Decel = ceil((J_MSR - LRL)*(RF/8)/Recovery_Time)
      | R_Accel = ceil((R_MSR - LRL)*RF/(Reaction_Time*10/60))
      | R_Decel = ceil((R_MSR - LRL)*(RF/8)/Recovery_Time)
      | }
  Steady -> Steady [order 2] : after(500, msec)[Activity >= Hys]
  Changes_Accelerations1 -> Walking_Accel
  Walking_Accel -> Changes_Accelerations1 [order 3] : after(500,msec)[MSR > Changing_Rate && Activity >= Hys]
  Starting_State -> Changes_Accelerations : after(200,msec)[Activity >= W_Thres]
  Changes_Accelerations -> Walking_Accel
  Walking_Accel -> Steady [order 2] : [Changing_Rate >= MSR]
  Walking_Decel -> Starting_State [order 2] : [Changing_Rate <= LRL]
  Walking_Accel -> Changes_To_Deceleration [order 1] : [Activity < Hys]
  Changes_To_Acceleration -> Walking_Accel
  Steady -> Walking_Decel [order 1] : [Activity < Hys]
  Changes_To_Deceleration -> Walking_Decel
  Walking_Decel -> Changes_To_Acceleration [order 1] : [Activity >= Thres]
  Changes_Decelerations -> Walking_Decel
  Walking_Decel -> Changes_Decelerations [order 3] : after(500,msec)[Changing_Rate > LRL && Activity < Hys]
  data: Activity input; LRL input uint16; RF input uint16; Reaction_Time input uint16; Recovery_Time input uint16; W_Thres input double; J_Thres input double; R_Thres input double; W_Hys input double; J_Hys input double; R_Hys input double; W_MSR input uint16; J_MSR input uint16; R_MSR input uint16; Changing_Rate output uint16; R_Accel local; R_Decel local; J_Accel local; J_Decel local; W_Accel local; W_Decel local; MSR input uint16; Accel local; Hys local; Thres local; Decel local

== stateflow chart simulink_A2_Final/Subsystem1/From DCM ==
  state Confirming_Values
    entry:
    DCM_SEND();
  state Default
    %general parameters
    MODE = uint8(6);
    LRL = uint16(60);
    URL = uint16(180);
    %AV_DELAY = 150;
    Reaction_Time = uint16(30);
    RF = uint16(16);
    W_Thres = double(0.5);
    J_Thres = double(1.75);
    R_Thres = double(3.0);
    Recovery_Time = uint16(5);
    W_MSR = uint16(80);
    J_MSR = uint16(120);
    R_MSR = uint16(160);
    W_Hys = double(0.75);
    J_Hys = double(1.75);
    R_Hys = double(2.75);
    %ATRIUM
    Atrium_Amp = single(3.0);
    ATR_Pulse_Width= uint16(1);
    A_Refractory_Period = uint16(250);
    ATR_Sense = single(4);
    %VENTRICLE
    Vent_Amp= single(3);
    Vent_Pulse_Width = uint16(1);
    V_Refractory_Period = uint16(200);
    VENT_Sense = single(4);
  state SET_PARAM
    entry:
    MODE = typecast(Rx(3), 'uint8')   ;
    LRL = typecast(Rx(4:5), 'uint16');
    URL = typecast(Rx(6:7), 'uint16');
    Reaction_Time  = typecast(Rx(8:9), 'uint16');
    RF = typecast(Rx(10:11), 'uint16');
    W_Thres = typecast(Rx(12:19), 'double');
    J_Thres = typecast(Rx(20:27), 'double');
    R_Thres = typecast(Rx(28:35), 'double');
    Recovery_Time = typecast(Rx(36:37), 'uint16');
    W_MSR = typecast(Rx(38:39), 'uint16');
    J_MSR = typecast(Rx(40:41), 'uint16');
    R_MSR = typecast(Rx(42:43), 'uint16');
    W_Hys = typecast(Rx(44:51), 'double');
    J_Hys = typecast(Rx(52:59), 'double');
    R_Hys = typecast(Rx(60:67), 'double');
    %ATR
    Atrium_Amp = typecast(Rx(68:71), 'single');
    ATR_Pulse_Width = typecast(Rx(72:73), 'uint16');
    A_Refractory_Period = typecast(Rx(74:75), 'uint16');
    ATR_Sense = typecast(Rx(76:79), 'single');
    %VENT
    Vent_Amp = typecast(Rx(80:83), 'single');
    Vent_Pulse_Width = typecast(Rx(84:85), 'uint16');
    V_Refractory_Period = typecast(Rx(86:87), 'uint16');
    VENT_Sense = typecast(Rx(88:91), 'single');
  state STANDBY
  state SEND_EGRAM
    entry:
    DCM_SEND();
  (default) -> Default
  SET_PARAM -> Confirming_Values : after(1000,msec)
  Confirming_Values -> STANDBY : after(1000,msec)
  (junction 7) -> STANDBY [order 2]
  Default -> STANDBY
  STANDBY -> (junction 7) : [Status == 0]
  (junction 7) -> (junction 10) [order 1] : [Rx(1) == hex2dec('00')]
  (junction 10) -> SET_PARAM [order 1] : [Rx(2) == hex2dec('00')]
  (junction 10) -> SEND_EGRAM [order 2] : [Rx(2) == hex2dec('01')]
  SEND_EGRAM -> STANDBY : after(1000,msec)
  data: LRL output uint16; Rx input uint8; Status input uint8; URL output uint16; MODE output uint8; Reaction_Time output uint16; RF output uint16; W_Thres output double; J_Thres output double; R_Thres output double; Recovery_Time output uint16; W_MSR output uint16; J_MSR output uint16; R_MSR output uint16; W_Hys output double; J_Hys output double; R_Hys output double; Atrium_Amp output single; ATR_Pulse_Width output uint16; A_Refractory_Period output uint16; ATR_Sense output single; Vent_Amp output single; Vent_Pulse_Width output uint16; V_Refractory_Period output uint16; VENT_Sense output single
